simulink model "Autopilot"  (R2019b)
settings: Solver=ode4  StartTime=Aircraft_Data.t_i  StopTime=Aircraft_Data.t_f  FixedStep=Aircraft_Data.dt  RelTol=1e-3
PostLoadFcn:
  | %% Adding File Path to MATLAb's Search Path
  | addpath(fileparts(which(bdroot)))
  | 
  | %% Aircraft Data
  | Data_From_Excel = readmatrix('B-747 Flight Condition 5.xlsx','Range','B2:B61');
  | Aircraft_Data = AircraftData(Data_From_Excel);
InitFcn:
  | %% Adding File Path to MATLAb's Search Path
  | addpath(fileparts(which(bdroot)))
  | 
  | %% Aircraft Data
  | Data_From_Excel = readmatrix('B-747 Flight Condition 5.xlsx','Range','B2:B61');
  | Aircraft_Data = AircraftData(Data_From_Excel);
libraries: simulink_extras x1
settings Model: Creator=Mahmoud A. Moustafa  LastModifiedBy=Mahmoud A. Moustafa

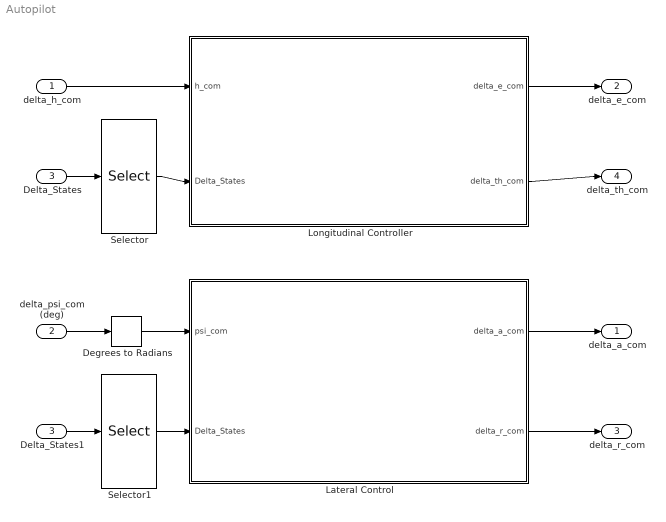
== system Autopilot ==
  delta_h_com : Inport  PortDimensions=1
  delta_psi_com (deg) : Inport  Port=2  PortDimensions=1
  Delta_States : Inport  Port=3  PortDimensions=18
  Degrees to Radians : simulink_extras/Transformations/Degrees to Radians
  Delta_States1 : InportShadow  Port=3  PortDimensions=18
  Lateral Control : Subsystem
  Longitudinal Controller : Subsystem
  Selector : Selector  InputPortWidth=18  IndexOptions=Index vector (dialog)  Indices=[7 11 5 3]  OutputSizes=1
  Selector1 : Selector  InputPortWidth=18  IndexOptions=Index vector (dialog)  Indices=[12 4 6]  OutputSizes=1
  delta_a_com : Outport  PortDimensions=1
  delta_e_com : Outport  Port=2  PortDimensions=1
  delta_r_com : Outport  Port=3  PortDimensions=1
  delta_th_com : Outport  Port=4  PortDimensions=1
  wires:
  delta_h_com/1 -> Longitudinal Controller/1(h_com)
  Delta_States/1 -> Selector/1
  Selector/1 -> Longitudinal Controller/2(Delta_States)
  Delta_States1/1 -> Selector1/1
  Longitudinal Controller/1(delta_e_com) -> delta_e_com/1
  Longitudinal Controller/2(delta_th_com) -> delta_th_com/1
  Selector1/1 -> Lateral Control/2(Delta_States)
  delta_psi_com (deg)/1 -> Degrees to Radians/1
  Lateral Control/1(delta_a_com) -> delta_a_com/1
  Lateral Control/2(delta_r_com) -> delta_r_com/1
  Degrees to Radians/1 -> Lateral Control/1(psi_com)

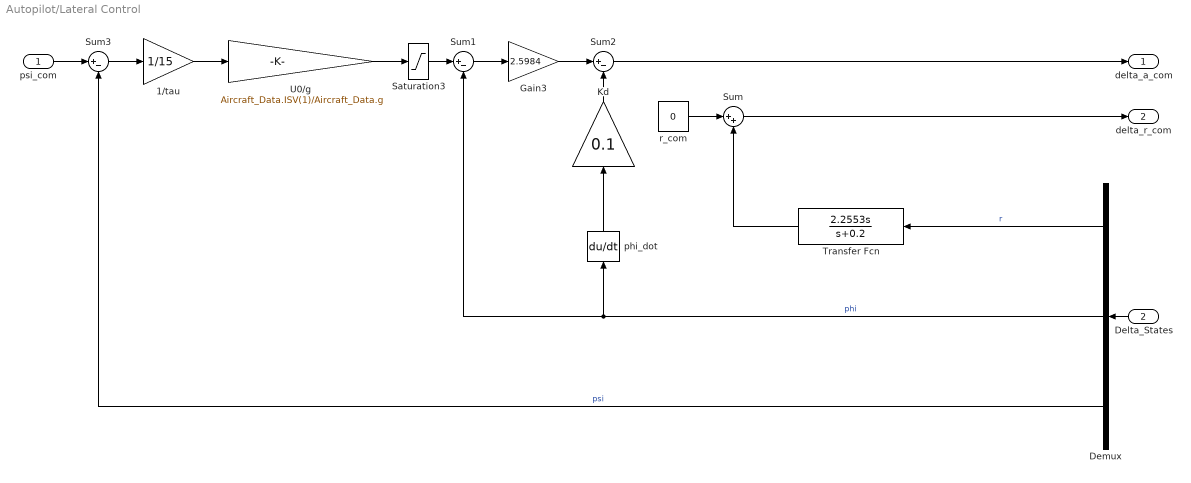
== system Autopilot/Lateral Control ==
  psi_com : Inport
  Delta_States : Inport  Port=2
  " Kd " : Gain  Gain=0.1
  "1/tau " : Gain  Gain=1/15
  Demux : Demux  Outputs=3
  Gain3 : Gain  Gain=2.5984
  Saturation3 : Saturate  UpperLimit=25*pi/180  LowerLimit=-25*pi/180
  Sum : Sum  Inputs=|++
  Sum1 : Sum  Inputs=|+-
  Sum2 : Sum  Inputs=|+-
  Sum3 : Sum  Inputs=|+-
  Transfer Fcn : TransferFcn  Numerator=[2.2553 0]  Denominator=[1 0.2]
  "U0/g " : Gain  Gain=Aircraft_Data.ISV(1)/Aircraft_Data.g
  "phi_dot " : Derivative  CoefficientInTFapproximation=0
  r_com : Constant  Value=0
  delta_a_com : Outport
  delta_r_com : Outport  Port=2
  wires:
  "phi_dot "/1 -> " Kd "/1
  Gain3/1 -> Sum2/1
  Demux/1 -> Transfer Fcn/1  "r"
  Demux/2 -> Sum1/2, "phi_dot "/1  "phi"
  Transfer Fcn/1 -> Sum/2
  Sum3/1 -> "1/tau "/1
  r_com/1 -> Sum/1
  Sum2/1 -> delta_a_com/1
  Sum1/1 -> Gain3/1
  "U0/g "/1 -> Saturation3/1
  Saturation3/1 -> Sum1/1
  psi_com/1 -> Sum3/1
  " Kd "/1 -> Sum2/2
  "1/tau "/1 -> "U0/g "/1
  Sum/1 -> delta_r_com/1
  Demux/3 -> Sum3/2  "psi"
  Delta_States/1 -> Demux/1

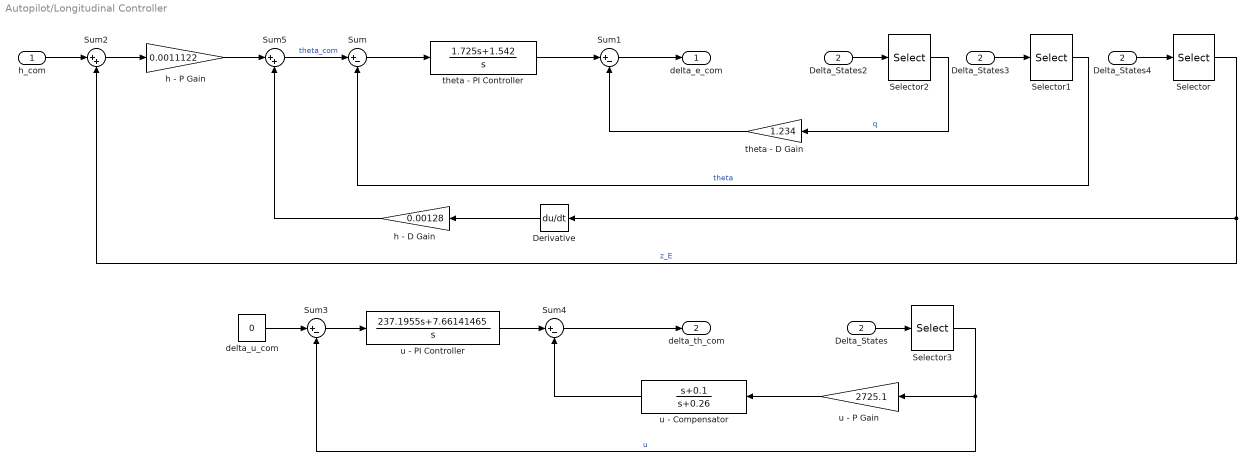
== system Autopilot/Longitudinal Controller ==
  h_com : Inport
  Delta_States : Inport  Port=2
  Delta_States2 : InportShadow  Port=2
  Delta_States3 : InportShadow  Port=2
  Delta_States4 : InportShadow  Port=2
  Derivative : Derivative
  Selector : Selector  InputPortWidth=4  IndexOptions=Index vector (dialog)  Indices=4  OutputSizes=1
  Selector1 : Selector  InputPortWidth=4  IndexOptions=Index vector (dialog)  Indices=3  OutputSizes=1
  Selector2 : Selector  InputPortWidth=4  IndexOptions=Index vector (dialog)  Indices=2  OutputSizes=1
  Selector3 : Selector  InputPortWidth=4  IndexOptions=Index vector (dialog)  Indices=1  OutputSizes=1
  Sum{,1,3..4} (4 alike) : Sum  Inputs=|+-
  Sum2 : Sum  Inputs=|++
  Sum5 : Sum  Inputs=|++
  delta_u_com : Constant  Value=0
  h - D Gain : Gain  Gain=0.00128
  h - P Gain : Gain  Gain=0.0011122
  theta - D Gain : Gain  Gain=1.234
  theta - PI Controller : TransferFcn  Numerator=[1.725 1.542]  Denominator=[1 0]
  u - Compensator : TransferFcn  Numerator=[1 0.1]  Denominator=[1 0.26]
  u - P Gain : Gain  Gain=2725.1
  u - PI Controller : TransferFcn  Numerator=[237.1955 7.66141465]  Denominator=[1 0]
  delta_e_com : Outport
  delta_th_com : Outport  Port=2
  wires:
  Sum3/1 -> u - PI Controller/1
  h - P Gain/1 -> Sum5/1
  Sum/1 -> theta - PI Controller/1
  Sum1/1 -> delta_e_com/1
  Sum2/1 -> h - P Gain/1
  Derivative/1 -> h - D Gain/1
  h - D Gain/1 -> Sum5/2
  Delta_States4/1 -> Selector/1
  h_com/1 -> Sum2/1
  Sum4/1 -> delta_th_com/1
  Sum5/1 -> Sum/1  "theta_com"
  Delta_States3/1 -> Selector1/1
  theta - PI Controller/1 -> Sum1/1
  theta - D Gain/1 -> Sum1/2
  u - PI Controller/1 -> Sum4/1
  u - Compensator/1 -> Sum4/2
  u - P Gain/1 -> u - Compensator/1
  delta_u_com/1 -> Sum3/1
  Delta_States/1 -> Selector3/1
  Selector/1 -> Derivative/1, Sum2/2  "z_E"
  Selector1/1 -> Sum/2  "theta"
  Delta_States2/1 -> Selector2/1
  Selector2/1 -> theta - D Gain/1  "q"
  Selector3/1 -> u - P Gain/1, Sum3/2  "u"
